simulink model "pendule_inv_etu"  (R2017a)
settings: Solver=VariableStepAuto  StartTime=0.0  StopTime=tf  RelTol=1e-3
values from neighbouring files (symbols this model uses):
  K = [30 10]    [exemple_test_pendule_inv.m]    (also in exemple_test_pendule_inv_capteur.m = [10 1]; exemple_test_pendule_inv_echant.m)
  x0 = [pi/10 0]    [exemple_test_pendule_inv.m]    (also in exemple_test_pendule_inv_capteur.m = [pi/20 0]; exemple_test_pendule_inv_echant.m = [pi/20 0])
settings Model: Creator=mkerrand  LastModifiedBy=mlarzul

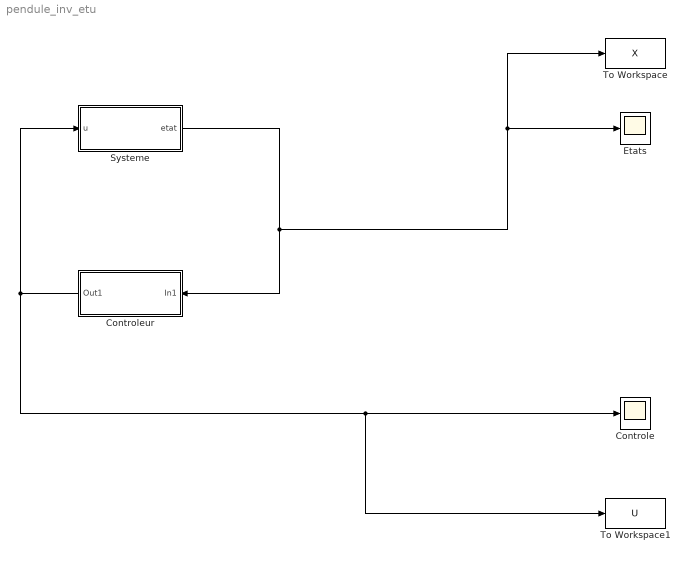
== system pendule_inv_etu ==
  Controle : Scope
  Controleur : Subsystem
  Etats : Scope
  Systeme : Subsystem
  To Workspace : ToWorkspace  VariableName=X  SaveFormat=Timeseries  SampleTime=-1
  To Workspace1 : ToWorkspace  VariableName=U  SaveFormat=Timeseries  SampleTime=-1
  wires:
  Controleur/1(Out1) -> To Workspace1/1, Controle/1, Systeme/1(u)
  Systeme/1("etat ") -> To Workspace/1, Etats/1, Controleur/1(In1)

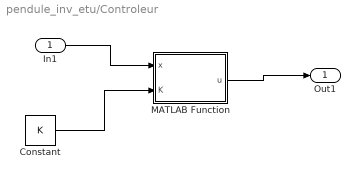
== system pendule_inv_etu/Controleur ==
  In1 : Inport
  Constant : Constant  Value=K
  MATLAB Function : MATLAB Function  TreatAsAtomicUnit=on
  Out1 : Outport
  wires:
  MATLAB Function/1(u) -> Out1/1
  In1/1 -> MATLAB Function/1(x)
  Constant/1 -> MATLAB Function/2(K)

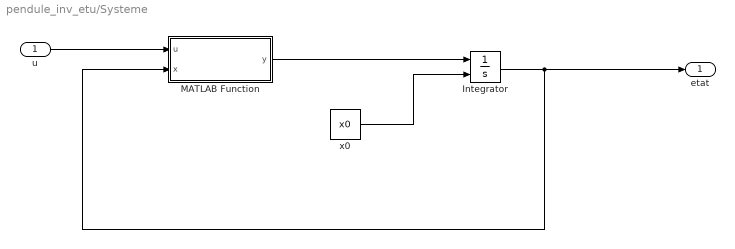
== system pendule_inv_etu/Systeme ==
  u : Inport
  Integrator : Integrator  InitialConditionSource=external
  MATLAB Function : MATLAB Function  TreatAsAtomicUnit=on
  x0 : Constant  Value=x0
  "etat " : Outport
  wires:
  u/1 -> MATLAB Function/1(u)
  MATLAB Function/1(y) -> Integrator/1
  Integrator/1 -> "etat "/1, MATLAB Function/2(x)
  x0/1 -> Integrator/2

== matlab function pendule_inv_etu/Systeme/MATLAB Function ==
  data: u input; y output; x input
function y = fcn(u,x)
    g=9.81;
    l=10;
        
    y1 = x(2);
    y2 = g/l*sin(x(1)) - (cos(x(1))*u)/l;
    y=[y1 y2]';

== matlab function pendule_inv_etu/Controleur/MATLAB Function ==
  data: x input; u output; K input
function u = fcn(x,K)
    
    xe = [0 0];
    ue = 0;
    
    u = ue + K'*(x-xe') ;
